simulink model "Phase1"  (R2016b)
settings: Solver=VariableStepAuto  StartTime=0.0  StopTime=40  RelTol=1e-3
settings Model: Creator=Sare  LastModifiedBy=Sare

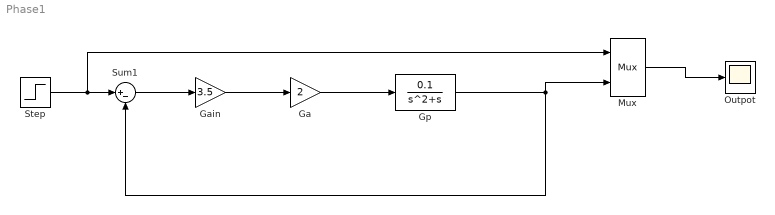
== system Phase1 ==
  Ga : Gain  Gain=2
  Gain : Gain  Gain=3.5
  Gp : TransferFcn  Numerator=[0.1]  Denominator=[1 1 0 ]
  Mux : Mux  Inputs=2
  Outpot : Scope
  Step : Step  After=4  SampleTime=0
  Sum1 : Sum  Inputs=|+-
  wires:
  Step/1 -> Mux/1, Sum1/1
  Mux/1 -> Outpot/1
  Gp/1 -> Sum1/2, Mux/2
  Sum1/1 -> Gain/1
  Gain/1 -> Ga/1
  Ga/1 -> Gp/1
